simulink model "w1prob9"  (R2020a)
settings: Solver=VariableStepAuto  StartTime=0.0  StopTime=10.0  RelTol=1e-3
settings Model: Creator=Anjali123  LastModifiedBy=Anjali123

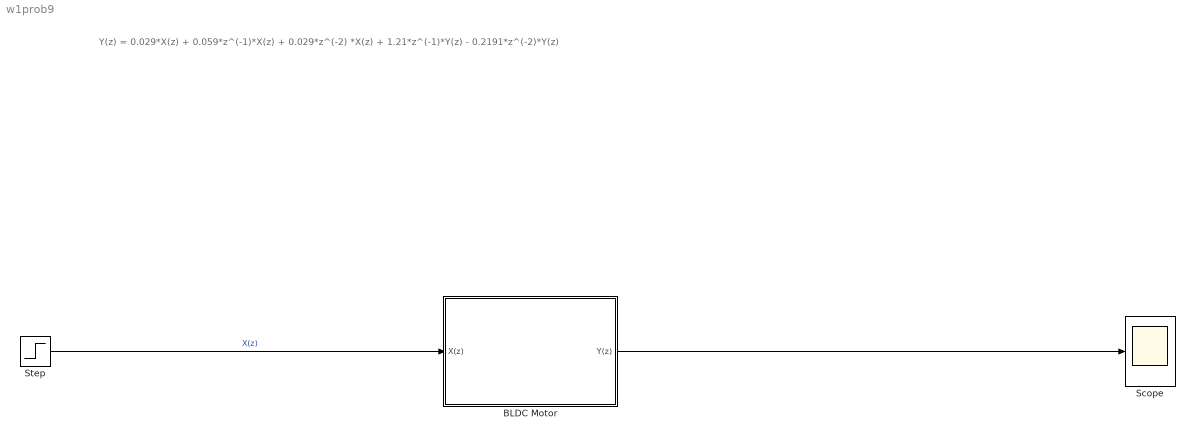
== system w1prob9 ==
  note: Y(z) = 0.029*X(z) + 0.059*z^(-1)*X(z) + 0.029*z^(-2) *X(z) + 1.21*z^(-1)*Y(z) - 0.2191*z^(-2)*Y(z)
  BLDC Motor : Subsystem
  Scope : Scope
  Step : Step  SampleTime=1/5000
  wires:
  Step/1 -> BLDC Motor/1(X(z))  "X(z)"
  BLDC Motor/1(Y(z)) -> Scope/1

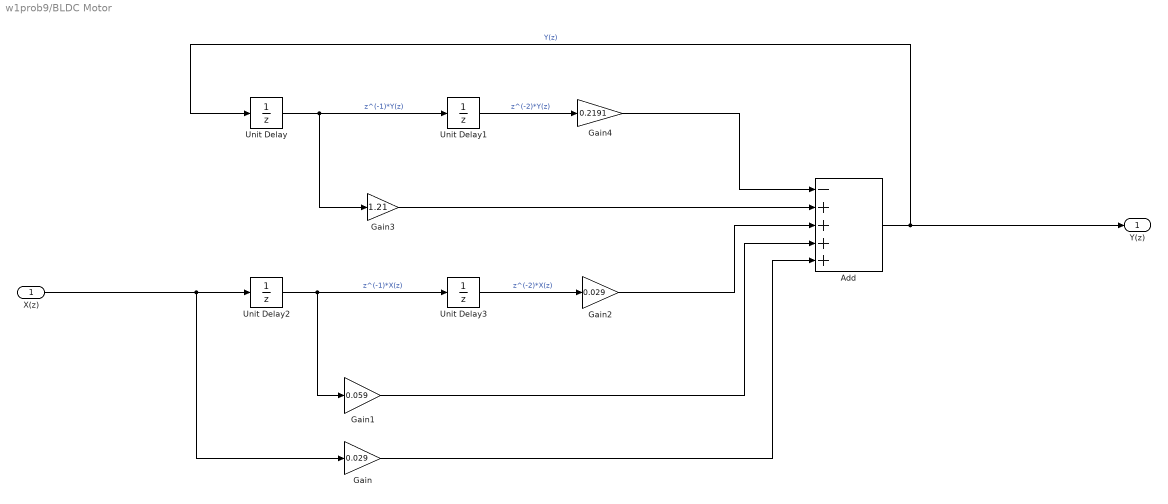
== system w1prob9/BLDC Motor ==
  X(z) : Inport
  Add : Sum  Inputs=-++++
  Gain : Gain  Gain=0.029
  Gain1 : Gain  Gain=0.059
  Gain2 : Gain  Gain=0.029
  Gain3 : Gain  Gain=1.21
  Gain4 : Gain  Gain=0.2191
  Unit Delay{,1..3} (4 alike) : UnitDelay  SampleTime=-1  HasFrameUpgradeWarning=on
  Y(z) : Outport
  wires:
  Unit Delay1/1 -> Gain4/1  "z^(-2)*Y(z)"
  Unit Delay3/1 -> Gain2/1  "z^(-2)*X(z)"
  Unit Delay/1 -> Gain3/1, Unit Delay1/1  "z^(-1)*Y(z)"
  Unit Delay2/1 -> Gain1/1, Unit Delay3/1  "z^(-1)*X(z)"
  X(z)/1 -> Gain/1, Unit Delay2/1
  Gain3/1 -> Add/2
  Gain2/1 -> Add/3
  Add/1 -> Y(z)/1, Unit Delay/1  "Y(z)"
  Gain/1 -> Add/5
  Gain1/1 -> Add/4
  Gain4/1 -> Add/1
